simulink model "compressor_as_scattered_LUP"  (R2023b)
settings: Solver=VariableStepAuto  StartTime=0.0  StopTime=10.0  RelTol=1e-3  AbsTol=1e-3
PreLoadFcn:
  | % Pressure ratio values in (Pa/Pa) obtained from reading a sample compresor data map
  | % Every row below corresponds to compressor map data for a RPM value that is chosen below
  | pressure_ratio = [1.2 1.18 1.16 1.14 1.12 1.1];
  | pressure_ratio = [pressure_ratio 1.48 1.44 1.40 1.36 1.32 1.28 1.24 1.2];
  | pressure_ratio = [pressure_ratio 1.8 1.75 1.7 1.65 1.6 1.55 1.50 1.45 1.4];
  | pressure_ratio = [pressure_ratio 2.2 2.1 2.0 1.9 1.8 1.75 1.70 1.65 1.6];
  | pressure_ratio = [pressure_ratio 2.6 2.5 2.4 2.3 2.2 2.1 2.0 1.9 1.8];
  | pressure_ratio = [pressure_ratio 3.02 3.01 3.00 2.9 2.8 2.7 2.6 2.5 2.4 2.24];
  | pressure_ratio = [pressure_ratio 3.6 3.59 3.58 3.5 3.4 3.3 3.2 3.1 3.0 2.9 2.8 2.7 2.6];
  | 
  | % Compressor RPM (length of every row corresponds to length of pressure_ratio values above)
  | rpm = [1500 1500 1500 1500 1500 1500];
  | rpm = [rpm 2000 2000 2000 2000 2000 2000 2000 2000];
  | rpm = [rpm 2500 2500 2500 2500 2500 2500 2500 2500 2500];
  | rpm = [rpm 3000 3000 3000 3000 3000 3000 3000 3000 3000];
  | rpm = [rpm 3500 3500 3500 3500 3500 3500 3500 3500 3500];
  | rpm = [rpm 4000 4000 4000 4000 4000 4000 4000 4000 4000 4000];
  | rpm = [rpm 4500 4500 4500 4500 4500 4500 4500 4500 4500 4500 4500 4500 4500];
  | 
  | % The mass flow rate values corresponding to the presure ratio and rpm values above
  | massflowrate = [0.4 0.6 0.85 1.05 1.4 1.6];
  | massflowrate = [massflowrate 0.7 0.8 1 1.4 1.6 2 2.3 2.6];
  | massflowrate = [massflowrate 1 1.5 2 2.5 2.75 2.8 3.2 3.4 3.6];
  | massflowrate = [massflowrate 1.2 2.2 2.8 3.1 3.3 3.5 4 4.1 4.2];
  | massflowrate = [massflowrate 1.8 2.8 3.2 3.6 4 4.2 4.6 4.8 5];
  | massflowrate = [massflowrate 2.2 2.6 3 4 4.4 4.6 4.8 5.1 5.3 5.7 ];
  | massflowrate = [massflowrate 2.9 3.1 3.4 4.3 4.8 5 5.2 5.5 5.6 5.7 5.8 5.9 6];
  | 
  | % A scaling factor applied on the RPM to ensure good triangulation for scatteredlookup.
  | % This factor is also applied at the input in the model
  | scaling_factor = 1000;
libraries: fl_lib x19, nesl_utility x4
CloseFcn:
  | try,close(h1_CompressorMapWithScatteredLookup),end
  | clear h1_CompressorMapWithScatteredLookup
  | 
  | clear tout simlog_CompressorMapWithScatteredLookup
  | clear pressure_ratio massflowrate rpm scaling_factor
Description:
  | Compressor Map with Scattered Lookup
settings Model: Creator=The MathWorks, Inc.  LastModifiedBy=kroblet
settings SolverCC: AutoScaleAbsTol=off  AlgebraicLoopSolver=TrustRegion  MaxZcPerStep=1
settings DataIOCC: ReturnWorkspaceOutputs=off
settings OptimizationCC: ReuseModelBlockBuffer=off
settings DebuggingCC: UnconnectedInputMsg=warning  UnconnectedOutputMsg=warning  UnconnectedLineMsg=warning  SymbolicDimsDataTypeCodeGenerationDiagnostic=none
settings ModelReferenceCC: EnableRefExpFcnMdlSchedulingChecks=on
settings SFSimCC: CustomCodeUndefinedFunction=UseInterfaceOnly
settings RTWCC: DLArmComputeVersion=19.05
settings SimscapeCC: SimscapeLogType=all  SimscapeLogSimulationStatistics=on  SimscapeLogName=simlog_CompressorMapWithScatteredLookup  SimscapeLogDataHistory=10000

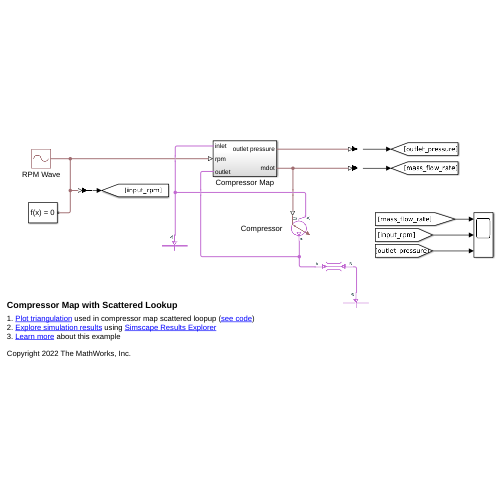
[thumbnail: Simulink's stored preview of the top-level diagram]
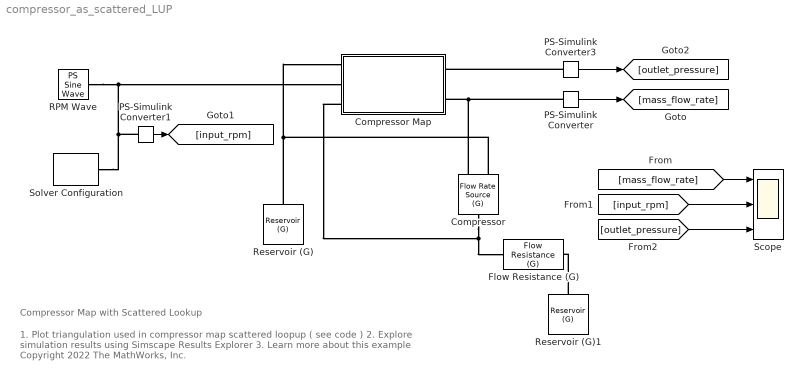
== system compressor_as_scattered_LUP ==
  note: Compressor Map with Scattered Lookup
  note: 1. Plot triangulation used in compressor map scattered loopup ( see code )
      | 2. Explore simulation results using Simscape Results Explorer
      | 3. Learn more about this example
      |
      | Copyright 2022 The MathWorks, Inc.
  Compressor : fl_lib/Gas/Sources/Flow Rate Source (G)  source_type=foundation.enum.constant_controlled.controlled  flow_type=foundation.enum.mass_volumetric_flow.mass  mass_flow=0 kg/s  volumetric_flow=0 m^3/s  volumetric_flow_conditions=foundation.enum.volumetric_flow_conditions.actual  p_std=0.101325 MPa  T_std=20 degC  power_spec=foundation.enum.power_spec.none  area_A=0.1 m^2  area_B=0.1 m^2
      settings: InternalSimscapePortConfiguration="{\"Bottom\":[],\"Left\":[{\"id\":\"A\",\"label\":\"A\",\"type\":\"foundation.gas.gas\"},{\"id\":\"M\",\"label\":\"M\",\"type\":\"input\"}],\"Right\":[{\"id\":\"B\",\"label\":\"B\",\"type\":\"foundation.gas.gas\"}],\"Top\":[]}"
  Compressor Map : Subsystem  Tag=PublishSubsystem
  Flow Resistance (G) : fl_lib/Gas/Elements/Flow Resistance (G)  delta_p_nominal=(2.0 - 1)*0.101325 MPa  mdot_nominal=3 kg/s  rho_nominal=0 kg/m^3  area=0.1 m^2  laminar_fraction=1e-3
      settings: InternalSimscapePortConfiguration="{\"Bottom\":[],\"Left\":[{\"id\":\"A\",\"label\":\"A\",\"type\":\"foundation.gas.gas\"}],\"Right\":[{\"id\":\"B\",\"label\":\"B\",\"type\":\"foundation.gas.gas\"}],\"Top\":[]}"
  PS-Simulink Converter : nesl_utility/PS-Simulink Converter  PhysicalDomain=network_engine_domain  SubClassName=ps_output  LeftPortType=input  RightPortType=output  PseudoPeriodic=off  Frequencies=[]  VectorFormat=inherit  Unit=kg/s  AffineConversion=off
  PS-Simulink Converter1 : nesl_utility/PS-Simulink Converter  PhysicalDomain=network_engine_domain  SubClassName=ps_output  LeftPortType=input  RightPortType=output  PseudoPeriodic=off  Frequencies=[]  VectorFormat=inherit  Unit=rpm  AffineConversion=off
  PS-Simulink Converter3 : nesl_utility/PS-Simulink Converter  PhysicalDomain=network_engine_domain  SubClassName=ps_output  LeftPortType=input  RightPortType=output  PseudoPeriodic=off  Frequencies=[]  VectorFormat=inherit  Unit=MPa  AffineConversion=off
  RPM Wave : fl_lib/Physical Signals/Sources/PS Sine Wave  amplitude=900 rpm  bias=3000 rpm  frequency_spec=foundation.enum.frequencySpec.frequencySI  frequency_SI=0.2 Hz  frequency_angular=1 rad/s  phase=0 rad
      settings: InternalSimscapePortConfiguration="{\"Bottom\":[],\"Left\":[],\"Right\":[{\"id\":\"O\",\"label\":\"\",\"type\":\"output\"}],\"Top\":[]}"
  Reservoir (G) : fl_lib/Gas/Elements/Reservoir (G)  pressure_spec=foundation.enum.pressure_spec.atmospheric  reservoir_pressure=0.101325 MPa  reservoir_temperature=288.15 K  area_A=0.1 m^2
  Reservoir (G)1 : fl_lib/Gas/Elements/Reservoir (G)  pressure_spec=foundation.enum.pressure_spec.atmospheric  reservoir_pressure=0.101325 MPa  reservoir_temperature=288.15 K  area_A=0.1 m^2
  Scope : Scope  NumInputPorts=3
  Solver Configuration : nesl_utility/Solver Configuration  PhysicalDomain=network_engine_domain  SubClassName=solver  LeftPortType=input  RightPortType=generic  Tones=[]  Harmonics=[]  SimulateNoise=off  Profile=off  UseLocalSampling=off  EnableSwitchedLinearOptims=on  FrequencyDomain=off  UseCCode=off  RelTol=0.001  AbsTol=0.001  MinStep=1e-09  ToWorkspace=off  RevertToSquareIcSolve=off  NumHomotopyIterations=100  PhasorMode=off  PhasorModeNumHarmonics=1  ConsistencySolver=NEWTON_XTOL_AFTER_FTOL  IndexReductionMethod=DerivativeReplacement  DoDC=off  ResidualTolerance=1e-09  ConsistencyTolSource=GLOBAL  ConsistencyAbsTol=0.001  ConsistencyRelTol=0.001  ConsistencyTolFactor=0.001  UseLocalSolver=off  LocalSolverChoice=NE_BACKWARD_EULER_ADVANCER  ResolveIndetEquations=on  FunctionEvalNumThread=1  LocalSolverSampleTime=0.001  DoFixedCost=off  MaxNonlinIter=3  MaxModeIter=2  ComputeImpulses=off  ImpulseIterations=2  LinearAlgebra=auto  LinearAlgebraNumThread=0  EquationFormulation=NE_TIME_EF  DelaysMemoryBudget=1024  AutomaticFiltering=on  FilteringTimeConstant=0.001  PartitionStorageMethod=AS_NEEDED  PartitionMemoryBudget=1024  PartitionMethod=ROBUST  MultibodyUseLocalSolver=off  MultibodyLocalSolverChoice=ODE1  MultibodyLocalSolverSampleTime=0.001
  wires:
  PS-Simulink Converter/1 -> [mass_flow_rate]
  PS-Simulink Converter3/1 -> [outlet_pressure]
  PS-Simulink Converter1/1 -> [input_rpm]
  [outlet_pressure] -> Scope/3
  [mass_flow_rate] -> Scope/1
  [input_rpm] -> Scope/2
  connections:
  Solver Configuration/RConn1 -- PS-Simulink Converter1/LConn1 -- RPM Wave/RConn1 -- Compressor Map/LConn2
  Reservoir (G)/LConn1 -- Compressor/LConn1 -- Compressor Map/LConn1
  Compressor/LConn2 -- Compressor Map/RConn2 -- PS-Simulink Converter/LConn1
  Compressor Map/LConn3 -- Flow Resistance (G)/LConn1 -- Compressor/RConn1
  PS-Simulink Converter3/LConn1 -- Compressor Map/RConn1
  Reservoir (G)1/LConn1 -- Flow Resistance (G)/RConn1

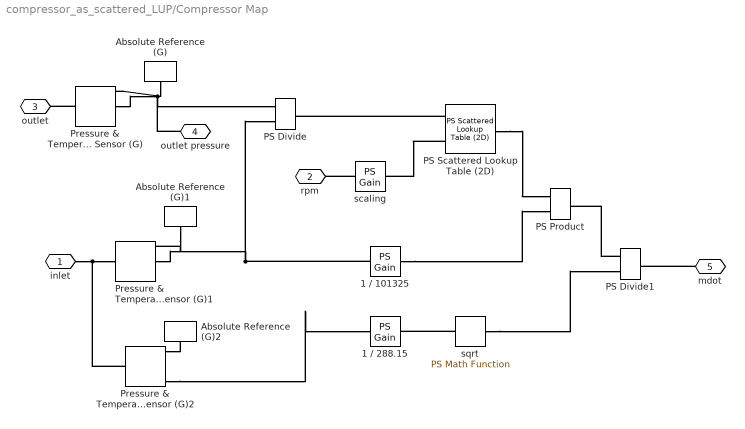
== system compressor_as_scattered_LUP/Compressor Map ==
  1 / 101325 : fl_lib/Physical Signals/Functions/PS Gain  gain=1/101325 1/Pa
  1 / 288.15 : fl_lib/Physical Signals/Functions/PS Gain  gain=1/288.15 1/K
  Absolute Reference (G) : fl_lib/Gas/Elements/Absolute Reference (G)
      settings: InternalSimscapePortConfiguration="{\"Bottom\":[],\"Left\":[{\"id\":\"A\",\"label\":\"\",\"type\":\"foundation.gas.gas\"}],\"Right\":[],\"Top\":[]}"
  Absolute Reference (G)1 : fl_lib/Gas/Elements/Absolute Reference (G)
      settings: InternalSimscapePortConfiguration="{\"Bottom\":[],\"Left\":[{\"id\":\"A\",\"label\":\"\",\"type\":\"foundation.gas.gas\"}],\"Right\":[],\"Top\":[]}"
  Absolute Reference (G)2 : fl_lib/Gas/Elements/Absolute Reference (G)
      settings: InternalSimscapePortConfiguration="{\"Bottom\":[],\"Left\":[{\"id\":\"A\",\"label\":\"\",\"type\":\"foundation.gas.gas\"}],\"Right\":[],\"Top\":[]}"
  PS Divide : fl_lib/Physical Signals/Functions/PS Divide
  PS Divide1 : fl_lib/Physical Signals/Functions/PS Divide
  PS Product : fl_lib/Physical Signals/Functions/PS Product
  PS Scattered Lookup Table (2D) : fl_lib/Physical Signals/Lookup Tables/PS Scattered Lookup Table (2D)  x1=pressure_ratio Pa/Pa  x2=rpm/scaling_factor rpm  f=massflowrate kg/s  extrap_method=simscape.enum.extrapolation_slu.nearest
      settings: InternalSimscapePortConfiguration="{\"Bottom\":[],\"Left\":[{\"id\":\"I1\",\"label\":\"x1\",\"type\":\"input\"},{\"id\":\"I2\",\"label\":\"x2\",\"type\":\"input\"}],\"Right\":[{\"id\":\"O\",\"label\":\"f\",\"type\":\"output\"}],\"Top\":[]}"
  Pressure & Temperature Sensor (G) : fl_lib/Gas/Sensors/Pressure & Temperature Sensor (G)  reference=foundation.enum.MeasurementReference.difference  pressure=true  pressure_spec=foundation.enum.PressureMeasementSpec.Absolute  temperature=true
      settings: InternalSimscapePortConfiguration="{\"Bottom\":[{\"id\":\"T\",\"label\":\"T\",\"type\":\"output\"}],\"Left\":[{\"id\":\"A\",\"label\":\"A\",\"type\":\"foundation.gas.gas\"}],\"Right\":[{\"id\":\"B\",\"label\":\"B\",\"type\":\"foundation.gas.gas\"},{\"id\":\"P\",\"label\":\"P\",\"type\":\"output\"}],\"Top\":[]}"
  Pressure & Temperature Sensor (G)1 : fl_lib/Gas/Sensors/Pressure & Temperature Sensor (G)  reference=foundation.enum.MeasurementReference.difference  pressure=true  pressure_spec=foundation.enum.PressureMeasementSpec.Absolute  temperature=true
      settings: InternalSimscapePortConfiguration="{\"Bottom\":[{\"id\":\"T\",\"label\":\"T\",\"type\":\"output\"}],\"Left\":[{\"id\":\"A\",\"label\":\"A\",\"type\":\"foundation.gas.gas\"}],\"Right\":[{\"id\":\"B\",\"label\":\"B\",\"type\":\"foundation.gas.gas\"},{\"id\":\"P\",\"label\":\"P\",\"type\":\"output\"}],\"Top\":[]}"
  Pressure & Temperature Sensor (G)2 : fl_lib/Gas/Sensors/Pressure & Temperature Sensor (G)  reference=foundation.enum.MeasurementReference.difference  pressure=true  pressure_spec=foundation.enum.PressureMeasementSpec.Absolute  temperature=true
      settings: InternalSimscapePortConfiguration="{\"Bottom\":[{\"id\":\"T\",\"label\":\"T\",\"type\":\"output\"}],\"Left\":[{\"id\":\"A\",\"label\":\"A\",\"type\":\"foundation.gas.gas\"}],\"Right\":[{\"id\":\"B\",\"label\":\"B\",\"type\":\"foundation.gas.gas\"},{\"id\":\"P\",\"label\":\"P\",\"type\":\"output\"}],\"Top\":[]}"
  scaling : fl_lib/Physical Signals/Functions/PS Gain  gain=1/1000
  sqrt : fl_lib/Physical Signals/Functions/PS Math Function  fcn_choice=foundation.enum.math_function.sqrt  v=1
  inlet : PMIOPort  Side=Left
  rpm : PMIOPort  Port=2  Side=Left
  outlet : PMIOPort  Port=3  Side=Left
  outlet pressure : PMIOPort  Port=4  Side=Right
  mdot : PMIOPort  Port=5  Side=Right
  connections:
  Pressure & Temperature Sensor (G)/LConn1 -- outlet/RConn1
  inlet/RConn1 -- Pressure & Temperature Sensor (G)2/LConn1 -- Pressure & Temperature Sensor (G)1/LConn1
  Pressure & Temperature Sensor (G)/RConn2 -- outlet pressure/RConn1 -- PS Divide/LConn1
  1 / 101325/LConn1 -- Pressure & Temperature Sensor (G)1/RConn2 -- PS Divide/LConn2
  PS Scattered Lookup Table (2D)/LConn1 -- PS Divide/RConn1
  PS Scattered Lookup Table (2D)/LConn2 -- scaling/RConn1
  Pressure & Temperature Sensor (G)2/RConn3 -- 1 / 288.15/LConn1
  PS Scattered Lookup Table (2D)/RConn1 -- PS Product/LConn1
  1 / 101325/RConn1 -- PS Product/LConn2
  PS Divide1/LConn1 -- PS Product/RConn1
  sqrt/RConn1 -- PS Divide1/LConn2
  mdot/RConn1 -- PS Divide1/RConn1
  sqrt/LConn1 -- 1 / 288.15/RConn1
  scaling/LConn1 -- rpm/RConn1
  Absolute Reference (G)/LConn1 -- Pressure & Temperature Sensor (G)/RConn1
  Absolute Reference (G)1/LConn1 -- Pressure & Temperature Sensor (G)1/RConn1
  Pressure & Temperature Sensor (G)2/RConn1 -- Absolute Reference (G)2/LConn1
